simulink model "system_dyninv_1st_order"  (R2018b)
settings: Solver=ode8  StartTime=0.0  StopTime=10  FixedStep=0.01  RelTol=1e-3
values from neighbouring files (symbols this model uses):
  A = -4    [dyninv_1st_order.m]
  B = 0.5    [dyninv_1st_order.m]
  C = 1    [dyninv_1st_order.m]
  CA = C*A    (= -4)    [dyninv_1st_order.m]
  invCB = inv(C*B)    [dyninv_1st_order.m]
  K = 2    [dyninv_1st_order.m]
settings Model: Creator=suvo.ganguli  LastModifiedBy=suvo.ganguli

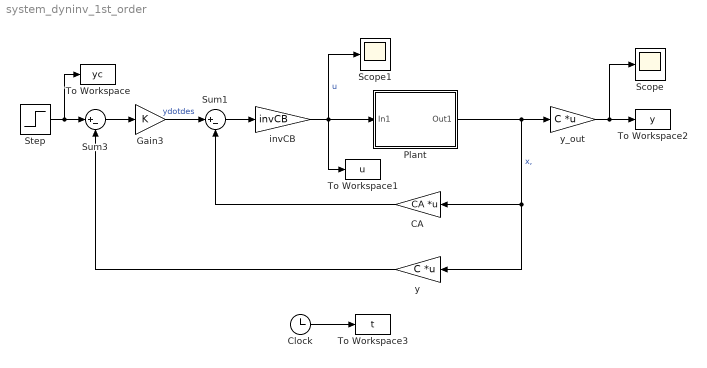
== system system_dyninv_1st_order ==
  CA : Gain  Gain=CA  Multiplication=Matrix(K*u)
  Clock : Clock
  Gain3 : Gain  Gain=K
  Plant : Subsystem
  Scope : Scope
  Scope1 : Scope
  Step : Step  SampleTime=0
  Sum1 : Sum  Inputs=|+-
  Sum3 : Sum  Inputs=|+-
  To Workspace : ToWorkspace  VariableName=yc  SampleTime=-1
  To Workspace1 : ToWorkspace  VariableName=u  SampleTime=-1
  To Workspace2 : ToWorkspace  VariableName=y  SampleTime=-1
  To Workspace3 : ToWorkspace  VariableName=t  SampleTime=-1
  invCB : Gain  Gain=invCB
  y : Gain  Gain=C  Multiplication=Matrix(K*u)
  y_out : Gain  Gain=C  Multiplication=Matrix(K*u)
  wires:
  Plant/1(Out1) -> y_out/1, y/1, CA/1  "x,"
  y/1 -> Sum3/2
  CA/1 -> Sum1/2
  y_out/1 -> To Workspace2/1, Scope/1
  Sum3/1 -> Gain3/1
  Step/1 -> To Workspace/1, Sum3/1
  Sum1/1 -> invCB/1
  invCB/1 -> To Workspace1/1, Scope1/1, Plant/1(In1)  "u"
  Gain3/1 -> Sum1/1  "ydotdes"
  Clock/1 -> To Workspace3/1

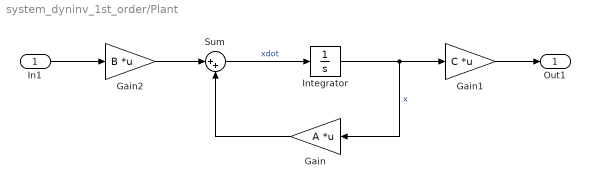
== system system_dyninv_1st_order/Plant ==
  In1 : Inport
  Gain : Gain  Gain=A  Multiplication=Matrix(K*u)
  Gain1 : Gain  Gain=C  Multiplication=Matrix(K*u)
  Gain2 : Gain  Gain=B  Multiplication=Matrix(K*u)
  Integrator : Integrator
  Sum : Sum  Inputs=|++
  Out1 : Outport
  wires:
  Integrator/1 -> Gain1/1, Gain/1  "x"
  Sum/1 -> Integrator/1  "xdot"
  Gain/1 -> Sum/2
  In1/1 -> Gain2/1
  Gain2/1 -> Sum/1
  Gain1/1 -> Out1/1
